simulink library "Lib_Cntrl_CorrectedGasFlow_TMATS"  (R2019b)
settings: Solver=ode45  StartTime=0.0  StopTime=10.0  RelTol=1e-3  EnableMultiTasking=on
Description:
  | Thomas Modules
settings Model: Creator=jwchapm2  LastModifiedBy=bhisma
settings DataIOCC: LimitDataPoints=on  SaveFormat=Array  ReturnWorkspaceOutputs=off
settings OptimizationCC: ExpressionDepthLimit=2147483647  LifeSpan=inf
settings DebuggingCC: UnderspecifiedInitializationDetection=Classic  MergeDetectMultiDrivingBlocksExec=none  SolverPrmCheckMsg=warning  StateNameClashWarn=warning  SFUnexpectedBacktrackingDiag=warning  SFNoUnconditionalDefaultTransitionDiag=warning  SFExecutionAtInitializationDiag=none  ArithmeticOperatorsInVariantConditions=warning
settings HardwareCC: ProdBitPerPointer=32  ProdBitPerSizeT=32  ProdBitPerPtrDiffT=32  ProdLargestAtomicFloat=None  ProdIntDivRoundTo=Undefined  ProdEndianess=Unspecified  ProdWordSize=32  ProdHWDeviceType=32-bit Generic
settings ModelReferenceCC: PropagateSignalLabelsOutOfModel=off
settings SFSimCC: SimUseLocalCustomCode=off  CustomCodeUndefinedFunction=UseInterfaceOnly
settings RTWCC: RTWUseLocalCustomCode=off
settings CodeAppCC: StateflowObjectComments=on
settings GRTTargetCC: TargetLangStandard=C89/C90 (ANSI)  GeneratePreprocessorConditionals=Disable all
settings ConfigComp: CovMetricSettings=dw  CovHtmlReporting=on  CovSaveCumulativeToWorkspaceVar=on  CovSaveSingleToWorkspaceVar=on  CovExternalEMLEnable=off

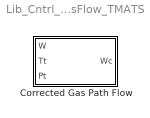
== system Lib_Cntrl_CorrectedGasFlow_TMATS ==
  Corrected Gas Path Flow : Subsystem  mask(T-MATS: Corrected Gas Path Flow Library Block){C_TSTD_M=518.67, C_PSTD_M=14.695951}
      mask prompts: C_TSTD_M "C_TSTD_M - Standard Day Temperature [degR]"; C_PSTD_M "C_PSTD_M - Standard Day Pressure [psia]"
      mask help:
      | This block calculates corrected flow.
      | Wc = W * sqrt(theta) /delta
      mask Help: web(which('Control_TMATS_CGPF.html'),'-helpbrowser')

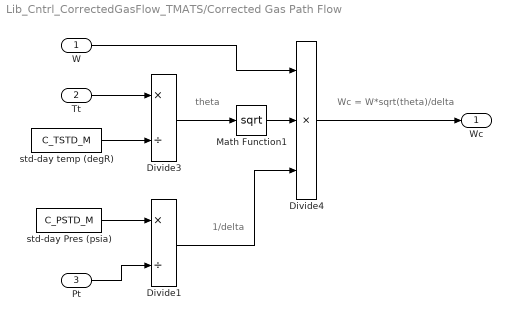
== system Lib_Cntrl_CorrectedGasFlow_TMATS/Corrected Gas Path Flow ==
  note: theta
  note: 1/delta
  note: Wc = W*sqrt(theta)/delta
  W : Inport
  Tt : Inport  Port=2
  Pt : Inport  Port=3
  Divide1 : Product  Inputs=*/
  Divide3 : Product  Inputs=*/
  Divide4 : Product  Inputs=***
  Math Function1 : Math  Operator=sqrt  SaturateOnIntegerOverflow=on
  std-day Pres (psia) : Constant  Value=C_PSTD_M
  std-day temp (degR) : Constant  Value=C_TSTD_M
  Wc : Outport
  wires:
  Tt/1 -> Divide3/1
  std-day temp (degR)/1 -> Divide3/2
  Divide3/1 -> Math Function1/1
  Math Function1/1 -> Divide4/2
  W/1 -> Divide4/1
  Divide4/1 -> Wc/1
  Divide1/1 -> Divide4/3
  std-day Pres (psia)/1 -> Divide1/1
  Pt/1 -> Divide1/2
